simulink library "battery_monitor_lib"  (R2022b)
settings: Solver=VariableStepAuto  StartTime=0.0  StopTime=10.0  RelTol=1e-3
settings Model: Creator=dr_pa  LastModifiedBy=dr_pa

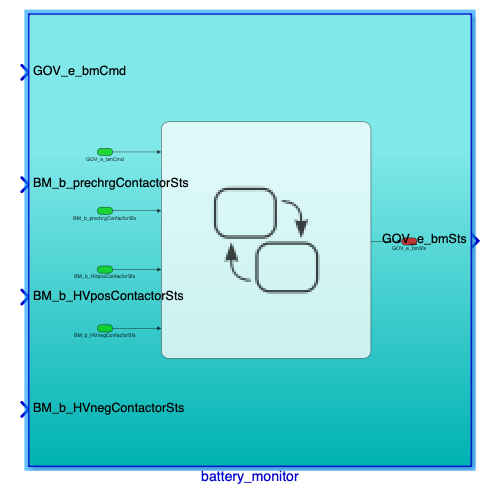
[thumbnail: Simulink's stored preview of the top-level diagram]
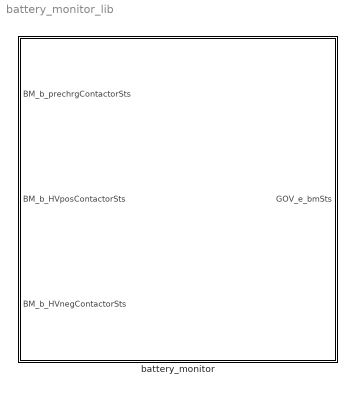
== system battery_monitor_lib ==
  battery_monitor : Subsystem

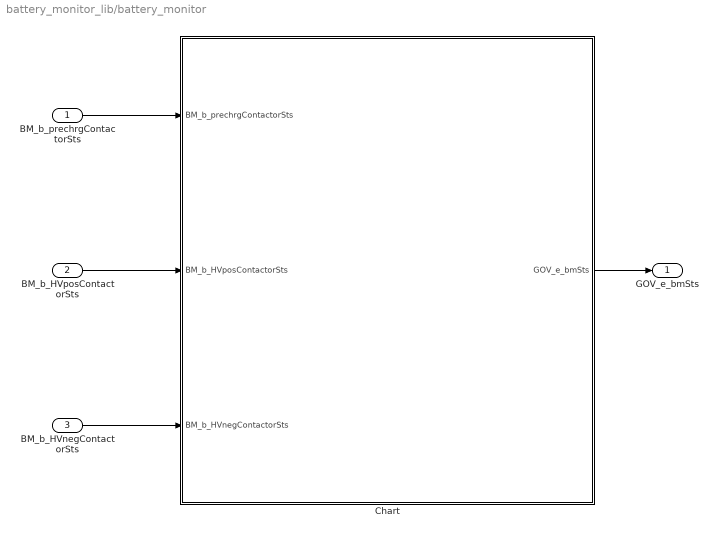
== system battery_monitor_lib/battery_monitor ==
  BM_b_prechrgContactorSts : Inport
  BM_b_HVposContactorSts : Inport  Port=2
  BM_b_HVnegContactorSts : Inport  Port=3
  Chart : Stateflow chart  TreatAsAtomicUnit=on
  GOV_e_bmSts : Outport
  wires:
  BM_b_prechrgContactorSts/1 -> Chart/1(BM_b_prechrgContactorSts)
  BM_b_HVposContactorSts/1 -> Chart/2(BM_b_HVposContactorSts)
  BM_b_HVnegContactorSts/1 -> Chart/3(BM_b_HVnegContactorSts)
  Chart/1(GOV_e_bmSts) -> GOV_e_bmSts/1

== stateflow chart battery_monitor_lib/battery_monitor/Chart ==
  state HV_connected
    en:
    GOV_e_bmSts = BM_STATUSES.RUNNING;
  state InitialState
    entry:
    GOV_e_bmSts = BM_STATUSES.INIT;
  state StartupState
    entry:
    GOV_BM_STATUS = STARTUP;
  state InitializePrechargeState
    entry:
    GOV_BM_STATUS = INIT_PRECHARGE;
  state PrechargeState
    entry:
    GOV_BM_STATUS = PRECHARGE;
  state RunningState
    entry:
    GOV_BM_STATUS = RUNNING;
  (default) -> InitialState
  InitialState -> HV_connected [order 2] : [(BM_b_prechrgContactorSts == 1) && ...
      | (BM_b_HVnegContactorSts == 1) && ...
      |  (BM_b_HVposContactorSts == 1)]
  InitialState -> StartupState [order 1] : [BM_b_prechrgContactorSts == 0 && BM_b_HVnegContactorSts == 0 && BM_b_HVposContactorSts == 0]
  StartupState -> InitializePrechargeState
  InitializePrechargeState -> PrechargeState
  PrechargeState -> RunningState
  data: BM_b_prechrgContactorSts input; BM_b_HVposContactorSts input; BM_b_HVnegContactorSts input; GOV_e_bmSts output Enum: BM_STATUSES; GOV_BM_STATUS local Enum: BM_STATUSES
